simulink model "pidControl"  (R2017b)
settings: Solver=ode4  StartTime=0.0  StopTime=10  FixedStep=1e-2  RelTol=1e-3
libraries: simulink x2
settings Model: Creator=Haotian  LastModifiedBy=Haotian

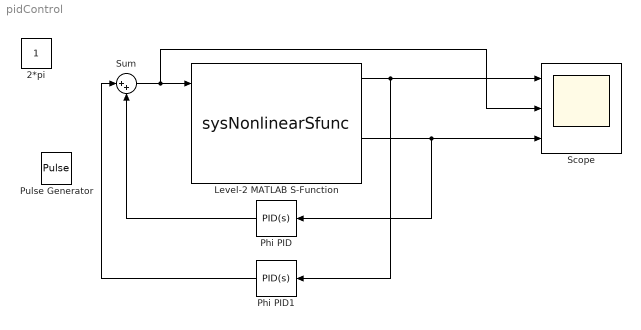
== system pidControl ==
  Level-2 MATLAB S-Function : M-S-Function  FunctionName=sysNonlinearSfunc  Parameters=Mc, Mg, b, l, I, init_phi, useAcc  mask(S-function: sysNonlinearSfunc){Mc=1.096, Mg=0.109, b=0.1, l=0.25, I=0.0034, init_phi=pi/10, useAcc=on}
      mask prompts: Mc "小车质量"; Mg "摆杆质量"; b "小车摩擦系数"; l "摆杆转动轴心到杆质心的长度"; I "摆杆惯量"; init_phi "初始垂直夹角"; useAcc "使用加速度作为输入"
      mask help: 一阶倒立摆非线性模型。
      mask Display:
      | fprintf('一阶倒立摆\n\nM=%.3f m=%.3f\nb=%.3f l=%.3f\nI=%.3f phi0=%.2f\n\nX=[x dx phi dphi]', Mc, Mg, b, l, I, init_phi);
      | if(useAcc)
      |     port_label('input', 1, 'a');
      | else
      |     port_label('input', 1, 'F');
      | end
      | port_label('input', 2, 'setX');
      | port_label('input', 3, 'devX');
      | 
      | port_label('output', 1, 'x');
      | port_label('output', 2, 'v');
      | port_label('output', 3, '\phi','texmode','on');
      | port_label('output', 4, 'd\phi','texmode','on');
  Phi PID : simulink/Continuous/PID Controller  Controller=PID  TimeDomain=Continuous-time  SampleTime=-1  IntegratorMethod=Forward Euler  FilterMethod=Forward Euler  Form=Parallel  UseFilter=on  ControllerParametersSource=internal  P=-40  I=0  D=-10  N=100  InitialConditionSource=internal  InitialConditionForIntegrator=0  InitialConditionForFilter=0  ExternalReset=none  LimitOutput=off  UpperSaturationLimit=inf  LowerSaturationLimit=-inf  LinearizeAsGain=on  AntiWindupMode=none  Kb=1  TrackingMode=off  Kt=1  PParamMin=[]  PParamMax=[]  IParamMin=[]  IParamMax=[]  DParamMin=[]  DParamMax=[]  NParamMin=[]  NParamMax=[]  KbParamMin=[]  KbParamMax=[]  KtParamMin=[]  KtParamMax=[]  POutMin=[]  POutMax=[]  IOutMin=[]  IOutMax=[]  DOutMin=[]  DOutMax=[]  NOutMin=[]  NOutMax=[]  KbOutMin=[]  KbOutMax=[]  KtOutMin=[]  KtOutMax=[]  IntegratorOutMin=[]  IntegratorOutMax=[]  FilterOutMin=[]  FilterOutMax=[]  SumOutMin=[]  SumOutMax=[]  SumI1OutMin=[]  SumI1OutMax=[]  SumI2OutMin=[]  SumI2OutMax=[]  SumI3OutMin=[]  SumI3OutMax=[]  SumDOutMin=[]  SumDOutMax=[]  SaturationOutMin=[]  SaturationOutMax=[]  IntegratorContinuousStateAttributes=''  IntegratorStateMustResolveToSignalObject=off  IntegratorRTWStateStorageClass=Auto  FilterContinuousStateAttributes=''  FilterStateMustResolveToSignalObject=off  FilterRTWStateStorageClass=Auto  DifferentiatorICPrevScaledInput=0  DifferentiatorOutMin=[]  DifferentiatorOutMax=[]  InitialConditionSetting=State (most efficient)  FilterDiffOutCoefMin=[]  FilterDiffOutCoefMax=[]  SumDenOutMin=[]  SumDenOutMax=[]  SumNumOutMin=[]  SumNumOutMax=[]  ReciprocalOutMin=[]  ReciprocalOutMax=[]  DivideOutMin=[]  DivideOutMax=[]  TunerSelectOption=Transfer Function Based (PID Tuner App)
  Phi PID1 : simulink/Continuous/PID Controller  Controller=PID  TimeDomain=Continuous-time  SampleTime=-1  IntegratorMethod=Forward Euler  FilterMethod=Forward Euler  Form=Parallel  UseFilter=on  ControllerParametersSource=internal  P=2  I=0.04  D=4.4  N=100  InitialConditionSource=internal  InitialConditionForIntegrator=0  InitialConditionForFilter=0  ExternalReset=none  LimitOutput=off  UpperSaturationLimit=inf  LowerSaturationLimit=-inf  LinearizeAsGain=on  AntiWindupMode=none  Kb=1  TrackingMode=off  Kt=1  PParamMin=[]  PParamMax=[]  IParamMin=[]  IParamMax=[]  DParamMin=[]  DParamMax=[]  NParamMin=[]  NParamMax=[]  KbParamMin=[]  KbParamMax=[]  KtParamMin=[]  KtParamMax=[]  POutMin=[]  POutMax=[]  IOutMin=[]  IOutMax=[]  DOutMin=[]  DOutMax=[]  NOutMin=[]  NOutMax=[]  KbOutMin=[]  KbOutMax=[]  KtOutMin=[]  KtOutMax=[]  IntegratorOutMin=[]  IntegratorOutMax=[]  FilterOutMin=[]  FilterOutMax=[]  SumOutMin=[]  SumOutMax=[]  SumI1OutMin=[]  SumI1OutMax=[]  SumI2OutMin=[]  SumI2OutMax=[]  SumI3OutMin=[]  SumI3OutMax=[]  SumDOutMin=[]  SumDOutMax=[]  SaturationOutMin=[]  SaturationOutMax=[]  IntegratorContinuousStateAttributes=''  IntegratorStateMustResolveToSignalObject=off  IntegratorRTWStateStorageClass=Auto  FilterContinuousStateAttributes=''  FilterStateMustResolveToSignalObject=off  FilterRTWStateStorageClass=Auto  DifferentiatorICPrevScaledInput=0  DifferentiatorOutMin=[]  DifferentiatorOutMax=[]  InitialConditionSetting=State (most efficient)  FilterDiffOutCoefMin=[]  FilterDiffOutCoefMax=[]  SumDenOutMin=[]  SumDenOutMax=[]  SumNumOutMin=[]  SumNumOutMax=[]  ReciprocalOutMin=[]  ReciprocalOutMax=[]  DivideOutMin=[]  DivideOutMax=[]  TunerSelectOption=Transfer Function Based (PID Tuner App)
  Pulse Generator : DiscretePulseGenerator  PulseType=Time based  Period=10  PhaseDelay=1
  Scope : Scope  NumInputPorts=3
  Sum : Sum  Inputs=|++
  2*pi : Constant  IOType=siggen
  wires:
  Level-2 MATLAB S-Function/1 -> Phi PID1/1, Scope/1
  Level-2 MATLAB S-Function/3 -> Phi PID/1, Scope/3
  Phi PID1/1 -> Sum/1
  Sum/1 -> Scope/2, Level-2 MATLAB S-Function/1
  Phi PID/1 -> Sum/2
